simulink model "Sim3Tanks_simulink"  (R2017a)
settings: Solver=ode45  StartTime=0  StopTime=400  FixedStep=0.1  RelTol=1e-3  EnableMultiTasking=on
PreLoadFcn:
  | try
  |     run('pre_settings')
  | catch
  |     for i = 1 : 3
  |         mainpath = dir('**/Sim3Tanks*.slx');
  |         if isempty(mainpath)
  |             cd('..');
  |         else
  |             run('simulink/simscripts/pre_settings')
  |             break;
  |         end
  |     end
  | end
InitFcn:
  | try
  |     run('simulink_settings')
  | catch
  |     for i = 1 : 3
  |         mainpath = dir('**/Sim3Tanks*.slx');
  |         if isempty(mainpath)
  |             cd('..');
  |         else
  |             run('simulink/simscripts/simulink_settings')
  |             break;
  |         end
  |     end
  | end
libraries: simulink x2
settings Model: Creator=AdministradorLAB  LastModifiedBy=AdminLab
settings DataIOCC: LimitDataPoints=on  SaveFormat=Array
settings OptimizationCC: LifeSpan=inf
settings DebuggingCC: UnderspecifiedInitializationDetection=Classic  MergeDetectMultiDrivingBlocksExec=none  SolverPrmCheckMsg=warning  SFUnexpectedBacktrackingDiag=warning  SFNoUnconditionalDefaultTransitionDiag=warning  SFExecutionAtInitializationDiag=none
settings HardwareCC: ProdBitPerPointer=32  ProdBitPerSizeT=32  ProdBitPerPtrDiffT=32  ProdLargestAtomicFloat=None  ProdIntDivRoundTo=Undefined  ProdEndianess=Unspecified  ProdWordSize=32  ProdHWDeviceType=32-bit Generic
settings ModelReferenceCC: PropagateSignalLabelsOutOfModel=off
settings GRTTargetCC: TargetLangStandard=C89/C90 (ANSI)  GeneratePreprocessorConditionals=Disable all
settings ConfigComp: CovMetricSettings=dw  CovHtmlReporting=on  CovSaveCumulativeToWorkspaceVar=on  CovSaveSingleToWorkspaceVar=on  CovExternalEMLEnable=off

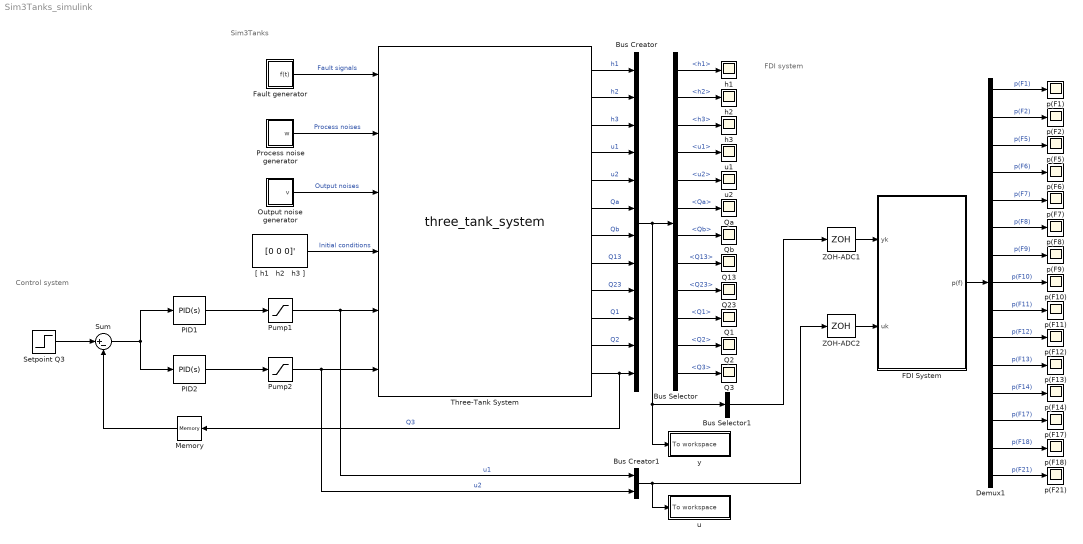
== system Sim3Tanks_simulink ==
  note: FDI system
  note: Control system
  note: Sim3Tanks
  Bus Creator : BusCreator  Inputs=12
  Bus Creator1 : BusCreator  Inputs=2
  Bus Selector : BusSelector  OutputSignals=h1,h2,h3,u1,u2,Qa,Qb,Q13,Q23,Q1,Q2,Q3
  Bus Selector1 : BusSelector  OutputSignals=h1,h2,h3,u1,u2,Q13,Q23,Q3  OutputAsBus=on
  Demux1 : Demux  Outputs=15
  FDI System : Subsystem
      mask Display:
      | disp('FDI system');
      | 
      | port_label('input',1,'yk');
      | port_label('input',2,'uk');
      | 
      | port_label('output',1,'p');
  Fault generator : Subsystem
      mask Display: port_label('output',1,'f');
  Memory : Memory
  Output noise generator : Subsystem
      mask Display: port_label('output',1,'v');
  PID1 : simulink/Continuous/PID Controller  Controller=PID  TimeDomain=Continuous-time  SampleTime=-1  IntegratorMethod=Forward Euler  FilterMethod=Forward Euler  Form=Parallel  UseFilter=on  ControllerParametersSource=internal  P=0.004  I=0.04  D=0.0001  N=100  InitialConditionSource=internal  InitialConditionForIntegrator=0  InitialConditionForFilter=0  ExternalReset=none  LimitOutput=off  UpperSaturationLimit=inf  LowerSaturationLimit=-inf  LinearizeAsGain=on  AntiWindupMode=none  Kb=1  TrackingMode=off  Kt=1  PParamMin=[]  PParamMax=[]  IParamMin=[]  IParamMax=[]  DParamMin=[]  DParamMax=[]  NParamMin=[]  NParamMax=[]  KbParamMin=[]  KbParamMax=[]  KtParamMin=[]  KtParamMax=[]  POutMin=[]  POutMax=[]  IOutMin=[]  IOutMax=[]  DOutMin=[]  DOutMax=[]  NOutMin=[]  NOutMax=[]  KbOutMin=[]  KbOutMax=[]  KtOutMin=[]  KtOutMax=[]  IntegratorOutMin=[]  IntegratorOutMax=[]  FilterOutMin=[]  FilterOutMax=[]  SumOutMin=[]  SumOutMax=[]  SumI1OutMin=[]  SumI1OutMax=[]  SumI2OutMin=[]  SumI2OutMax=[]  SumI3OutMin=[]  SumI3OutMax=[]  SumDOutMin=[]  SumDOutMax=[]  SaturationOutMin=[]  SaturationOutMax=[]  IntegratorContinuousStateAttributes=''  IntegratorStateMustResolveToSignalObject=off  IntegratorRTWStateStorageClass=Auto  FilterContinuousStateAttributes=''  FilterStateMustResolveToSignalObject=off  FilterRTWStateStorageClass=Auto  DifferentiatorICPrevScaledInput=0  DifferentiatorOutMin=[]  DifferentiatorOutMax=[]  InitialConditionSetting=State (most efficient)
  PID2 : simulink/Continuous/PID Controller  Controller=PID  TimeDomain=Continuous-time  SampleTime=-1  IntegratorMethod=Forward Euler  FilterMethod=Forward Euler  Form=Parallel  UseFilter=on  ControllerParametersSource=internal  P=0.004  I=0.04  D=0.0001  N=100  InitialConditionSource=internal  InitialConditionForIntegrator=0  InitialConditionForFilter=0  ExternalReset=none  LimitOutput=off  UpperSaturationLimit=inf  LowerSaturationLimit=-inf  LinearizeAsGain=on  AntiWindupMode=none  Kb=1  TrackingMode=off  Kt=1  PParamMin=[]  PParamMax=[]  IParamMin=[]  IParamMax=[]  DParamMin=[]  DParamMax=[]  NParamMin=[]  NParamMax=[]  KbParamMin=[]  KbParamMax=[]  KtParamMin=[]  KtParamMax=[]  POutMin=[]  POutMax=[]  IOutMin=[]  IOutMax=[]  DOutMin=[]  DOutMax=[]  NOutMin=[]  NOutMax=[]  KbOutMin=[]  KbOutMax=[]  KtOutMin=[]  KtOutMax=[]  IntegratorOutMin=[]  IntegratorOutMax=[]  FilterOutMin=[]  FilterOutMax=[]  SumOutMin=[]  SumOutMax=[]  SumI1OutMin=[]  SumI1OutMax=[]  SumI2OutMin=[]  SumI2OutMax=[]  SumI3OutMin=[]  SumI3OutMax=[]  SumDOutMin=[]  SumDOutMax=[]  SaturationOutMin=[]  SaturationOutMax=[]  IntegratorContinuousStateAttributes=''  IntegratorStateMustResolveToSignalObject=off  IntegratorRTWStateStorageClass=Auto  FilterContinuousStateAttributes=''  FilterStateMustResolveToSignalObject=off  FilterRTWStateStorageClass=Auto  DifferentiatorICPrevScaledInput=0  DifferentiatorOutMin=[]  DifferentiatorOutMax=[]  InitialConditionSetting=State (most efficient)
  Process noise generator : Subsystem
      mask Display: port_label('output',1,'w');
  Pump1 : Saturate  UpperLimit=80  LowerLimit=0
  Pump2 : Saturate  UpperLimit=80  LowerLimit=0
  Q{1..3,13,23} (5 alike) : Scope
  Qa : Scope
  Qb : Scope
  Setpoint Q3 : Step  Time=0  After=120  SampleTime=0.1
  Sum : Sum  Inputs=|+-
  Three-Tank System : M-S-Function  FunctionName=three_tank_system  mask{editTs=0.1, editRR=5, editHmax=50, editR=0.635, edith0=30, editmi=1, editg=981, cboxKp1=on, cboxKp2=on, cboxKa=off, cboxKb=off, cboxK13=on, cboxK23=on, cboxK1=off, cboxK3=on, cboxK2=off, cboxOpen=on, cboxClosed=off, cboxFromWS=off, f1mag=0, f1type=Stepwise, f1start=150, f1stop=300, f2mag=0, f2type=Stepwise, f2start=150, f2stop=300, f3mag=0, f3type=Stepwise, f3start=150, f3stop=300, f4mag=0, f4type=Stepwise, f4start=150, f4stop=300, f5mag=0, f5type=Stepwise, f5start=150, f5stop=300, f6mag=0, f6type=Stepwise, f6start=150, f6stop=300, f7mag=0, f7type=Stepwise, f7start=150, f7stop=300, f8mag=0, f8type=Stepwise, f8start=150, f8stop=300, f9mag=0, f9type=Stepwise, f9start=150, f9stop=300, f10mag=0, f10type=Stepwise, f10start=150, f10stop=300, f11mag=0, f11type=Stepwise, f11start=150, f11stop=300, f12mag=0, f12type=Stepwise, f12start=150, f12stop=300, f13mag=0, f13type=Stepwise, f13start=150, f13stop=300, f14mag=0, f14type=Stepwise, f14start=150, f14stop=300, f15mag=0, f15type=Stepwise, f15start=150, f15stop=300, f16mag=0, f16type=Stepwise, f16start=150, f16stop=300, f17mag=0, f17type=Stepwise, f17start=150, f17stop=300, f18mag=0, f18type=Stepwise, f18start=150, f18stop=300, f19mag=0, f19type=Stepwise, f19start=150, f19stop=300, f20mag=0, f20type=Stepwise, f20start=150, f20stop=300, f21mag=0, f21type=Stepwise, f21start=150, f21stop=300}
      mask prompts: editRR "Tanks radius (cm):"; editHmax "Tanks height (cm):"; editR "Pipes radius (cm):"; edith0 "Transmission pipes height (cm):"; editmi "Flow correction term (-):"; editg "Gravity constant (cm/s^2):"; cboxKp1 "Kp1"; cboxKp2 "Kp2"; cboxKa "Ka"; cboxKb "Kb"; cboxK13 "K13"; cboxK23 "K23"; cboxK1 "K1"; cboxK3 "K3"; cboxK2 "K2"; cboxOpen "Open"; cboxClosed "Closed"; cboxFromWS "From workspace"; f1type "Type:"; f1start "Start time:"; f1stop "Stop time:"; f2type "Type:"; f2start "Start time:"; f2stop "Stop time:"; f3type "Type:"; f3start "Start time:"; f3stop "Stop time:"; f4type "Type:"; f4start "Start time:"; f4stop "Stop time:"; f5type "Type:"; f5start "Start time:"; f5stop "Stop time:"; f6type "Type:"; f6start "Start time:"; f6stop "Stop time:"; f7type "Type:"; f7start "Start time:"; f7stop "Stop time:"; f8type "Type:"; f8start "Start time:"; f8stop "Stop time:"; f9type "Type:"; f9start "Start time:"; f9stop "Stop time:"; f10type "Type:"; f10start "Start time:"; f10stop "Stop time:"; f11type "Type:"; f11start "Start time:"; f11stop "Stop time:"; f12type "Type:"; f12start "Start time:"; f12stop "Stop time:"; f13type "Type:"; f13start "Start time:"; f13stop "Stop time:"; f14type "Type:"; f14start "Start time:"; f14stop "Stop time:"; f15type "Type:"; f15start "Start time:"; f15stop "Stop time:"; f16type "Type:"; f16start "Start time:"; f16stop "Stop time:"; f17type "Type:"; f17start "Start time:"; f17stop "Stop time:"; f18type "Type:"; f18start "Start time:"; f18stop "Stop time:"; f19type "Type:"; f19start "Start time:"; f19stop "Stop time:"; f20type "Type:"; f20start "Start time:"; f20stop "Stop time:"; f21type "Type:"; f21start "Start time:"; f21stop "Stop time:"
      mask Help: eval('gui_help_simulink');
      mask Callback cboxFromWS:
      | try
      |     run('from_workspace');
      | catch
      |     for i = 1 : 3
      |         mainpath = dir('**/Sim3Tanks*.slx');
      |         if isempty(mainpath)
      |             cd('..');
      |         else
      |             run('simulink/simscripts/from_workspace');
      |             break;
      |         end
      |     end
      | end
      mask TypeOptions f1type: Stepwise | Driftwise
      mask TypeOptions f2type: Stepwise | Driftwise
      mask TypeOptions f3type: Stepwise | Driftwise
      mask TypeOptions f4type: Stepwise | Driftwise
      mask TypeOptions f5type: Stepwise | Driftwise
      mask TypeOptions f6type: Stepwise | Driftwise
      mask TypeOptions f7type: Stepwise | Driftwise
      mask TypeOptions f8type: Stepwise | Driftwise
      mask TypeOptions f9type: Stepwise | Driftwise
      mask TypeOptions f10type: Stepwise | Driftwise
      mask TypeOptions f11type: Stepwise | Driftwise
      mask TypeOptions f12type: Stepwise | Driftwise
      mask TypeOptions f13type: Stepwise | Driftwise
      mask TypeOptions f14type: Stepwise | Driftwise
      mask TypeOptions f15type: Stepwise | Driftwise
      mask TypeOptions f16type: Stepwise | Driftwise
      mask TypeOptions f17type: Stepwise | Driftwise
      mask TypeOptions f18type: Stepwise | Driftwise
      mask TypeOptions f19type: Stepwise | Driftwise
      mask TypeOptions f20type: Stepwise | Driftwise
      mask TypeOptions f21type: Stepwise | Driftwise
      mask DialogControl txt1 Prompt: Tanks:
      mask DialogControl txt2 Prompt: Tank 1
      mask DialogControl txt3 Prompt: Tank 3
      mask DialogControl txt4 Prompt: Tank 2
      mask DialogControl txt5 Prompt: Pumps valves:
      mask DialogControl txt6 Prompt: --
      mask DialogControl txt7 Prompt: Transmission valves:
      mask DialogControl txt8 Prompt: --
      mask DialogControl txt9 Prompt: Connection valves:
      mask DialogControl txt10 Prompt: --
      mask DialogControl txt11 Prompt: Output valves:
      mask DialogControl hlink Prompt: Edit the fault signals in "/simulink/fault_signals.m"
      mask DialogControl hlink Callback: open('fault_signals');
      mask Display:
      | disp('Sim3Tanks');
      | 
      | port_label('input',1,'f');
      | port_label('input',2,'w');
      | port_label('input',3,'v');
      | port_label('input',4,'hi');
      | port_label('input',5,'u1');
      | port_label('input',6,'u2');
      | 
      | port_label('output',1,'y1');
      | port_label('output',2,'y2');
      | port_label('output',3,'y3');
      | port_label('output',4,'y4');
      | port_label('output',5,'y5');
      | port_label('output',6,'y6');
      | port_label('output',7,'y7');
      | port_label('output',8,'y8');
      | port_label('output',9,'y9');
      | port_label('output',10,'y10');
      | port_label('output',11,'y11');
      | port_label('output',12,'y12');
  ZOH-ADC1 : ZeroOrderHold  SampleTime=0.1
  ZOH-ADC2 : ZeroOrderHold  SampleTime=0.1
  "[ h1   h2   h3 ]" : Constant  Value=[0 0 0]'  SampleTime=0.1
  h1 : Scope
  h2 : Scope
  h3 : Scope
  p(F1) : Scope
  p(F10) : Scope
  p(F11) : Scope
  p(F12) : Scope
  p(F13) : Scope
  p(F14) : Scope
  p(F17) : Scope
  p(F18) : Scope
  p(F2) : Scope
  p(F21) : Scope
  p(F5) : Scope
  p(F6) : Scope
  p(F7) : Scope
  p(F8) : Scope
  p(F9) : Scope
  u : Subsystem
      mask Display: disp('To workspace');
  u1 : Scope
  u2 : Scope
  y : Subsystem
      mask Display: disp('To workspace');
  wires:
  "[ h1   h2   h3 ]"/1 -> Three-Tank System/4  "Initial conditions"
  Fault generator/1(f(t)) -> Three-Tank System/1  "Fault signals"
  Process noise generator/1(w) -> Three-Tank System/2  "Process noises"
  Output noise generator/1(v) -> Three-Tank System/3  "Output noises"
  Setpoint Q3/1 -> Sum/1
  Pump1/1 -> Bus Creator1/1, Three-Tank System/5  "u1"
  Memory/1 -> Sum/2
  Pump2/1 -> Bus Creator1/2, Three-Tank System/6  "u2"
  PID2/1 -> Pump2/1
  PID1/1 -> Pump1/1
  Sum/1 -> PID2/1, PID1/1
  Three-Tank System/1 -> Bus Creator/1  "h1"
  Three-Tank System/2 -> Bus Creator/2  "h2"
  Three-Tank System/3 -> Bus Creator/3  "h3"
  Three-Tank System/4 -> Bus Creator/4  "u1"
  Three-Tank System/5 -> Bus Creator/5  "u2"
  Three-Tank System/6 -> Bus Creator/6  "Qa"
  Three-Tank System/7 -> Bus Creator/7  "Qb"
  Three-Tank System/8 -> Bus Creator/8  "Q13"
  Three-Tank System/9 -> Bus Creator/9  "Q23"
  Three-Tank System/10 -> Bus Creator/10  "Q1"
  Three-Tank System/11 -> Bus Creator/11  "Q2"
  Three-Tank System/12 -> Memory/1, Bus Creator/12  "Q3"
  Bus Creator/1 -> Bus Selector/1, y/1(To workspace), Bus Selector1/1
  Bus Selector/1 -> h1/1  "<h1>"
  Bus Selector/2 -> h2/1  "<h2>"
  Bus Selector/3 -> h3/1  "<h3>"
  Bus Selector/4 -> u1/1  "<u1>"
  Bus Selector/5 -> u2/1  "<u2>"
  Bus Selector/6 -> Qa/1  "<Qa>"
  Bus Selector/7 -> Qb/1  "<Qb>"
  Bus Selector/8 -> Q13/1  "<Q13>"
  Bus Selector/9 -> Q23/1  "<Q23>"
  Bus Selector/10 -> Q1/1  "<Q1>"
  Bus Selector/11 -> Q2/1  "<Q2>"
  Bus Selector/12 -> Q3/1  "<Q3>"
  Bus Selector1/1 -> ZOH-ADC1/1
  Bus Creator1/1 -> u/1(To workspace), ZOH-ADC2/1
  Demux1/1 -> p(F1)/1  "p(F1)"
  Demux1/2 -> p(F2)/1  "p(F2)"
  Demux1/3 -> p(F5)/1  "p(F5)"
  Demux1/4 -> p(F6)/1  "p(F6)"
  Demux1/5 -> p(F7)/1  "p(F7)"
  Demux1/6 -> p(F8)/1  "p(F8)"
  Demux1/7 -> p(F9)/1  "p(F9)"
  Demux1/8 -> p(F10)/1  "p(F10)"
  Demux1/9 -> p(F11)/1  "p(F11)"
  Demux1/10 -> p(F12)/1  "p(F12)"
  Demux1/11 -> p(F13)/1  "p(F13)"
  Demux1/12 -> p(F14)/1  "p(F14)"
  Demux1/13 -> p(F17)/1  "p(F17)"
  Demux1/14 -> p(F18)/1  "p(F18)"
  Demux1/15 -> p(F21)/1  "p(F21)"
  ZOH-ADC1/1 -> FDI System/1(yk)
  ZOH-ADC2/1 -> FDI System/2(uk)
  FDI System/1(p(f)) -> Demux1/1

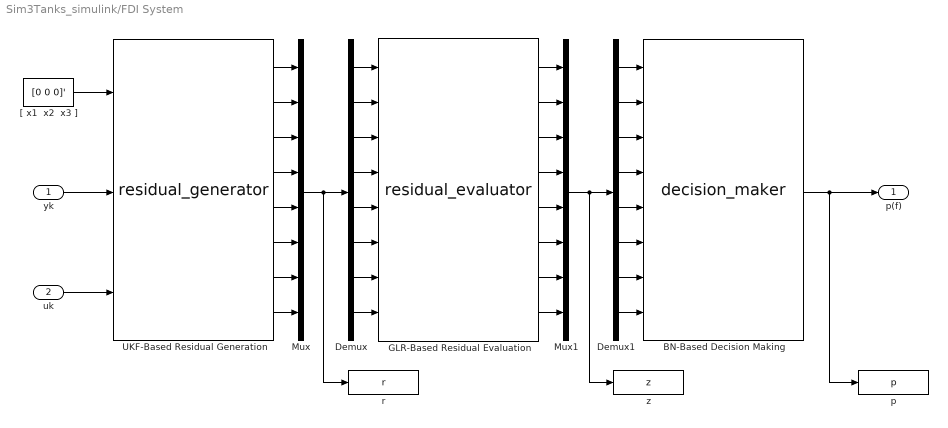
== system Sim3Tanks_simulink/FDI System ==
  yk : Inport
  uk : Inport  Port=2
  BN-Based Decision Making : M-S-Function  FunctionName=decision_maker
      mask Display:
      | disp('Decision Maker');
      | 
      | port_label('input',1,'z1');
      | port_label('input',2,'z2');
      | port_label('input',3,'z3');
      | port_label('input',4,'z4');
      | port_label('input',5,'z5');
      | port_label('input',6,'z6');
      | port_label('input',7,'z7');
      | port_label('input',8,'z8');
      | 
      | port_label('output',1,'p');
  Demux : Demux  Outputs=8
  Demux1 : Demux  Outputs=8
  GLR-Based Residual Evaluation : M-S-Function  FunctionName=residual_evaluator
      mask Display:
      | disp('Residual Evaluator');
      | 
      | port_label('input',1,'r1');
      | port_label('input',2,'r2');
      | port_label('input',3,'r3');
      | port_label('input',4,'r4');
      | port_label('input',5,'r5');
      | port_label('input',6,'r6');
      | port_label('input',7,'r7');
      | port_label('input',8,'r8');
      | 
      | port_label('output',1,'z1');
      | port_label('output',2,'z2');
      | port_label('output',3,'z3');
      | port_label('output',4,'z4');
      | port_label('output',5,'z5');
      | port_label('output',6,'z6');
      | port_label('output',7,'z7');
      | port_label('output',8,'z8');
  Mux : Mux  Inputs=8
  Mux1 : Mux  Inputs=8
  UKF-Based Residual Generation : M-S-Function  FunctionName=residual_generator
      mask Display:
      | disp('Residual Generator');
      | 
      | port_label('input',1,'xhat0');
      | port_label('input',2,'yk');
      | port_label('input',3,'uk');
      | 
      | port_label('output',1,'h1 => r1');
      | port_label('output',2,'h2 => r2');
      | port_label('output',3,'h3 => r3');
      | port_label('output',4,'u1 => r4');
      | port_label('output',5,'u2 => r5');
      | port_label('output',6,'Q13 => r6');
      | port_label('output',7,'Q23 => r7');
      | port_label('output',8,'Q3 => r8');
  "[ x1  x2  x3 ]" : Constant  Value=[0 0 0]'  SampleTime=0.1
  p : ToWorkspace  VariableName=p  SaveFormat=Timeseries  SampleTime=-1
      mask Display: disp('To workspace');
  r : ToWorkspace  VariableName=r  SaveFormat=Timeseries  SampleTime=-1
      mask Display: disp('To workspace');
  z : ToWorkspace  VariableName=z  SaveFormat=Timeseries  SampleTime=-1
      mask Display: disp('To workspace');
  p(f) : Outport
  wires:
  UKF-Based Residual Generation/2 -> Mux/2
  UKF-Based Residual Generation/5 -> Mux/5
  UKF-Based Residual Generation/8 -> Mux/8
  UKF-Based Residual Generation/4 -> Mux/4
  UKF-Based Residual Generation/1 -> Mux/1
  UKF-Based Residual Generation/3 -> Mux/3
  UKF-Based Residual Generation/6 -> Mux/6
  UKF-Based Residual Generation/7 -> Mux/7
  Mux/1 -> r/1, Demux/1
  "[ x1  x2  x3 ]"/1 -> UKF-Based Residual Generation/1
  uk/1 -> UKF-Based Residual Generation/3
  yk/1 -> UKF-Based Residual Generation/2
  Demux/1 -> GLR-Based Residual Evaluation/1
  Demux/2 -> GLR-Based Residual Evaluation/2
  Demux/3 -> GLR-Based Residual Evaluation/3
  Demux/4 -> GLR-Based Residual Evaluation/4
  Demux/5 -> GLR-Based Residual Evaluation/5
  Demux/6 -> GLR-Based Residual Evaluation/6
  Demux/7 -> GLR-Based Residual Evaluation/7
  Demux/8 -> GLR-Based Residual Evaluation/8
  GLR-Based Residual Evaluation/1 -> Mux1/1
  GLR-Based Residual Evaluation/2 -> Mux1/2
  GLR-Based Residual Evaluation/3 -> Mux1/3
  GLR-Based Residual Evaluation/4 -> Mux1/4
  GLR-Based Residual Evaluation/5 -> Mux1/5
  GLR-Based Residual Evaluation/6 -> Mux1/6
  GLR-Based Residual Evaluation/7 -> Mux1/7
  GLR-Based Residual Evaluation/8 -> Mux1/8
  Demux1/1 -> BN-Based Decision Making/1
  Demux1/2 -> BN-Based Decision Making/2
  Demux1/3 -> BN-Based Decision Making/3
  Demux1/4 -> BN-Based Decision Making/4
  Demux1/5 -> BN-Based Decision Making/5
  Demux1/6 -> BN-Based Decision Making/6
  Demux1/7 -> BN-Based Decision Making/7
  Demux1/8 -> BN-Based Decision Making/8
  Mux1/1 -> z/1, Demux1/1
  BN-Based Decision Making/1 -> p(f)/1, p/1

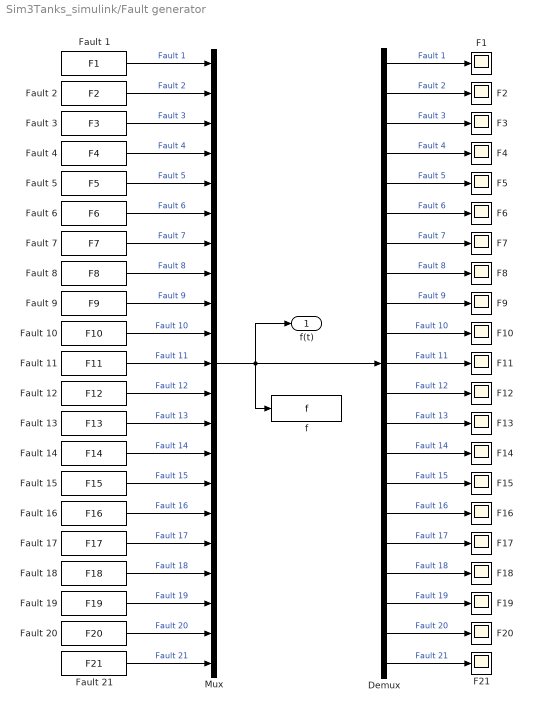
== system Sim3Tanks_simulink/Fault generator ==
  Demux : Demux  Outputs=21
  F{1..21} (21 alike) : Scope
  Fault 1 : FromWorkspace  VariableName=F1  SampleTime=0.1
  Fault 10 : FromWorkspace  VariableName=F10  SampleTime=0.1
  Fault 11 : FromWorkspace  VariableName=F11  SampleTime=0.1
  Fault 12 : FromWorkspace  VariableName=F12  SampleTime=0.1
  Fault 13 : FromWorkspace  VariableName=F13  SampleTime=0.1
  Fault 14 : FromWorkspace  VariableName=F14  SampleTime=0.1
  Fault 15 : FromWorkspace  VariableName=F15  SampleTime=0.1
  Fault 16 : FromWorkspace  VariableName=F16  SampleTime=0.1
  Fault 17 : FromWorkspace  VariableName=F17  SampleTime=0.1
  Fault 18 : FromWorkspace  VariableName=F18  SampleTime=0.1
  Fault 19 : FromWorkspace  VariableName=F19  SampleTime=0.1
  Fault 2 : FromWorkspace  VariableName=F2  SampleTime=0.1
  Fault 20 : FromWorkspace  VariableName=F20  SampleTime=0.1
  Fault 21 : FromWorkspace  VariableName=F21  SampleTime=0.1
  Fault 3 : FromWorkspace  VariableName=F3  SampleTime=0.1
  Fault 4 : FromWorkspace  VariableName=F4  SampleTime=0.1
  Fault 5 : FromWorkspace  VariableName=F5  SampleTime=0.1
  Fault 6 : FromWorkspace  VariableName=F6  SampleTime=0.1
  Fault 7 : FromWorkspace  VariableName=F7  SampleTime=0.1
  Fault 8 : FromWorkspace  VariableName=F8  SampleTime=0.1
  Fault 9 : FromWorkspace  VariableName=F9  SampleTime=0.1
  Mux : Mux  Inputs=21
  f : ToWorkspace  VariableName=f  SaveFormat=Timeseries  SampleTime=-1
      mask Display: disp('To workspace');
  f(t) : Outport
  wires:
  Fault 1/1 -> Mux/1  "Fault 1"
  Fault 2/1 -> Mux/2  "Fault 2"
  Fault 3/1 -> Mux/3  "Fault 3"
  Fault 4/1 -> Mux/4  "Fault 4"
  Fault 5/1 -> Mux/5  "Fault 5"
  Fault 6/1 -> Mux/6  "Fault 6"
  Fault 7/1 -> Mux/7  "Fault 7"
  Fault 8/1 -> Mux/8  "Fault 8"
  Fault 9/1 -> Mux/9  "Fault 9"
  Fault 10/1 -> Mux/10  "Fault 10"
  Fault 11/1 -> Mux/11  "Fault 11"
  Fault 12/1 -> Mux/12  "Fault 12"
  Fault 13/1 -> Mux/13  "Fault 13"
  Fault 14/1 -> Mux/14  "Fault 14"
  Fault 15/1 -> Mux/15  "Fault 15"
  Fault 16/1 -> Mux/16  "Fault 16"
  Fault 17/1 -> Mux/17  "Fault 17"
  Fault 18/1 -> Mux/18  "Fault 18"
  Fault 19/1 -> Mux/19  "Fault 19"
  Fault 20/1 -> Mux/20  "Fault 20"
  Fault 21/1 -> Mux/21  "Fault 21"
  Mux/1 -> f(t)/1, Demux/1, f/1
  Demux/1 -> F1/1  "Fault 1"
  Demux/2 -> F2/1  "Fault 2"
  Demux/3 -> F3/1  "Fault 3"
  Demux/4 -> F4/1  "Fault 4"
  Demux/5 -> F5/1  "Fault 5"
  Demux/6 -> F6/1  "Fault 6"
  Demux/7 -> F7/1  "Fault 7"
  Demux/8 -> F8/1  "Fault 8"
  Demux/9 -> F9/1  "Fault 9"
  Demux/10 -> F10/1  "Fault 10"
  Demux/11 -> F11/1  "Fault 11"
  Demux/12 -> F12/1  "Fault 12"
  Demux/13 -> F13/1  "Fault 13"
  Demux/14 -> F14/1  "Fault 14"
  Demux/15 -> F15/1  "Fault 15"
  Demux/16 -> F16/1  "Fault 16"
  Demux/17 -> F17/1  "Fault 17"
  Demux/18 -> F18/1  "Fault 18"
  Demux/19 -> F19/1  "Fault 19"
  Demux/20 -> F20/1  "Fault 20"
  Demux/21 -> F21/1  "Fault 21"

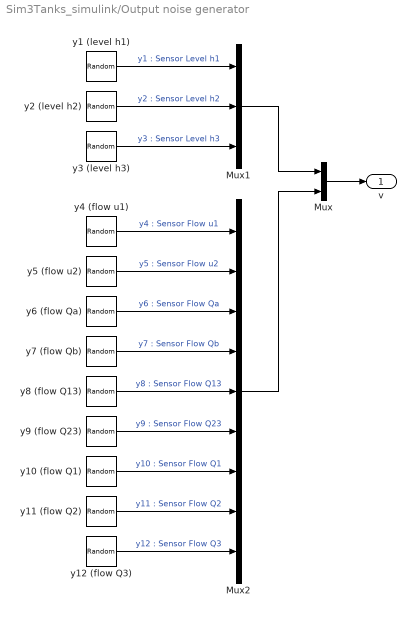
== system Sim3Tanks_simulink/Output noise generator ==
  Mux : Mux  Inputs=2
  Mux1 : Mux  Inputs=3
  Mux2 : Mux  Inputs=9
  y1 (level h1) : RandomNumber  Variance=0.01  SampleTime=0.1
  y10 (flow Q1) : RandomNumber  Variance=0.5  SampleTime=0.1
  y11 (flow Q2) : RandomNumber  Variance=0.5  SampleTime=0.1
  y12 (flow Q3) : RandomNumber  Variance=0.5  SampleTime=0.1
  y2 (level h2) : RandomNumber  Variance=0.01  SampleTime=0.1
  y3 (level h3) : RandomNumber  Variance=0.01  SampleTime=0.1
  y4 (flow u1) : RandomNumber  Variance=0.5  SampleTime=0.1
  y5 (flow u2) : RandomNumber  Variance=0.5  SampleTime=0.1
  y6 (flow Qa) : RandomNumber  Variance=0.5  SampleTime=0.1
  y7 (flow Qb) : RandomNumber  Variance=0.5  SampleTime=0.1
  y8 (flow Q13) : RandomNumber  Variance=0.5  SampleTime=0.1
  y9 (flow Q23) : RandomNumber  Variance=0.5  SampleTime=0.1
  v : Outport
  wires:
  y2 (level h2)/1 -> Mux1/2  "y2 : Sensor Level h2"
  y3 (level h3)/1 -> Mux1/3  "y3 : Sensor Level h3"
  y4 (flow u1)/1 -> Mux2/1  "y4 : Sensor Flow u1"
  y5 (flow u2)/1 -> Mux2/2  "y5 : Sensor Flow u2"
  y6 (flow Qa)/1 -> Mux2/3  "y6 : Sensor Flow Qa"
  y7 (flow Qb)/1 -> Mux2/4  "y7 : Sensor Flow Qb"
  y8 (flow Q13)/1 -> Mux2/5  "y8 : Sensor Flow Q13"
  y9 (flow Q23)/1 -> Mux2/6  "y9 : Sensor Flow Q23"
  y10 (flow Q1)/1 -> Mux2/7  "y10 : Sensor Flow Q1"
  y11 (flow Q2)/1 -> Mux2/8  "y11 : Sensor Flow Q2"
  y12 (flow Q3)/1 -> Mux2/9  "y12 : Sensor Flow Q3"
  y1 (level h1)/1 -> Mux1/1  "y1 : Sensor Level h1"
  Mux1/1 -> Mux/1
  Mux2/1 -> Mux/2
  Mux/1 -> v/1

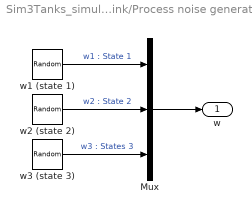
== system Sim3Tanks_simulink/Process noise generator ==
  Mux : Mux  Inputs=3
  w1 (state 1) : RandomNumber  Variance=0.0  SampleTime=0.1
  w2 (state 2) : RandomNumber  Variance=0.0  SampleTime=0.1
  w3 (state 3) : RandomNumber  Variance=0.0  SampleTime=0.1
  w : Outport
  wires:
  Mux/1 -> w/1
  w1 (state 1)/1 -> Mux/1  "w1 : State 1"
  w2 (state 2)/1 -> Mux/2  "w2 : State 2"
  w3 (state 3)/1 -> Mux/3  "w3 : States 3"

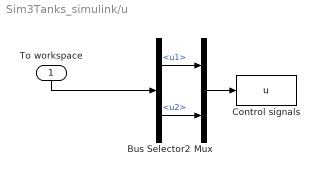
== system Sim3Tanks_simulink/u ==
  To workspace : Inport
  Bus Selector2 : BusSelector  OutputSignals=u1,u2
  Control signals : ToWorkspace  VariableName=u  SaveFormat=Timeseries  SampleTime=-1
  Mux : Mux  Inputs=2
  wires:
  Bus Selector2/2 -> Mux/2  "<u2>"
  Bus Selector2/1 -> Mux/1  "<u1>"
  To workspace/1 -> Bus Selector2/1
  Mux/1 -> Control signals/1

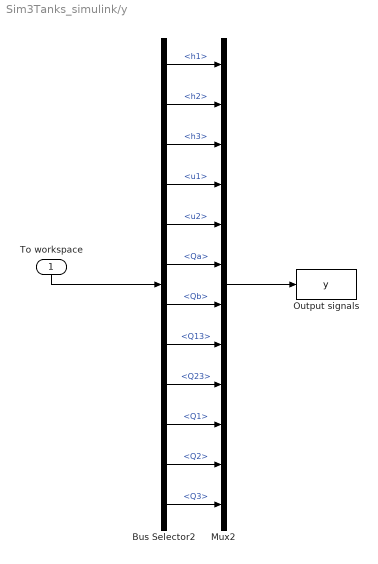
== system Sim3Tanks_simulink/y ==
  To workspace : Inport
  Bus Selector2 : BusSelector  OutputSignals=h1,h2,h3,u1,u2,Qa,Qb,Q13,Q23,Q1,Q2,Q3
  Mux2 : Mux  Inputs=12
  Output signals : ToWorkspace  VariableName=y  SaveFormat=Timeseries  SampleTime=-1
  wires:
  Mux2/1 -> Output signals/1
  Bus Selector2/7 -> Mux2/7  "<Qb>"
  Bus Selector2/9 -> Mux2/9  "<Q23>"
  Bus Selector2/4 -> Mux2/4  "<u1>"
  Bus Selector2/3 -> Mux2/3  "<h3>"
  Bus Selector2/5 -> Mux2/5  "<u2>"
  Bus Selector2/6 -> Mux2/6  "<Qa>"
  Bus Selector2/8 -> Mux2/8  "<Q13>"
  Bus Selector2/10 -> Mux2/10  "<Q1>"
  Bus Selector2/1 -> Mux2/1  "<h1>"
  Bus Selector2/11 -> Mux2/11  "<Q2>"
  Bus Selector2/12 -> Mux2/12  "<Q3>"
  Bus Selector2/2 -> Mux2/2  "<h2>"
  To workspace/1 -> Bus Selector2/1
